simulink model "ball_and_beam"  (R2020b)
settings: Solver=VariableStepAuto  StartTime=0.0  StopTime=10.0  RelTol=1e-3
values from neighbouring files (symbols this model uses):
  h = 0.01    [main_ball_and_beam_dlqr.m]
  setpoint = -0.5    [main_ball_and_beam_dlqr.m]
  X0 = [0; 0; 0; 0]    [main_ball_and_beam_dlqr.m]
undefined symbols (not defined in the file or in its folder): add_states, lstates, ubar, xbar
libraries: cstblocks x1
settings Model: Creator=Kingdel  LastModifiedBy=mluser

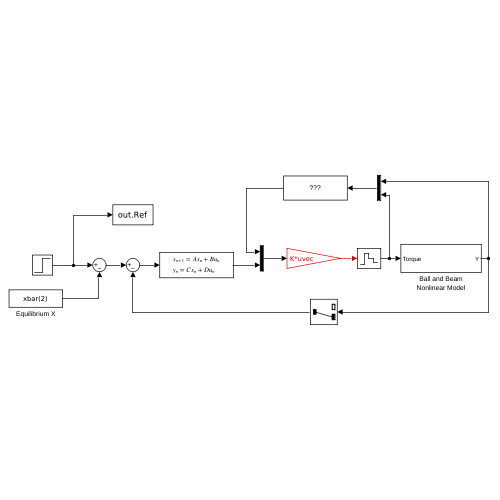
[thumbnail: Simulink's stored preview of the top-level diagram]
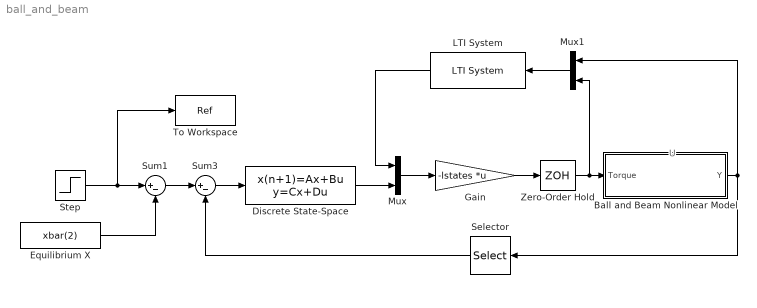
== system ball_and_beam ==
  note: U
  Ball and Beam Nonlinear Model : Subsystem
  Discrete State-Space : DiscreteStateSpace  A=add_states.A  B=add_states.B  C=eye(size(add_states.A))  D=zeros(size(add_states.B))  SampleTime=h
  Equilibrium X : Constant  Value=xbar(2)
  Gain : Gain  Gain=-lstates  Multiplication=Matrix(K*u) (u vector)  SampleTime=h
  LTI System : cstblocks/LTI System  sys=observer  IC=[]
  Mux : Mux  Inputs=2
  Mux1 : Mux  Inputs=2
  Selector : Selector  InputPortWidth=2  IndexOptions=Index vector (dialog)  Indices=2  OutputSizes=1
  Step : Step  Time=0  After=setpoint  SampleTime=h
  Sum1 : Sum  Inputs=|+-
  Sum3 : Sum  Inputs=|+-
  To Workspace : ToWorkspace  VariableName=Ref  SaveFormat=Structure With Time  SampleTime=h
  Zero-Order Hold : ZeroOrderHold  SampleTime=h
  wires:
  Gain/1 -> Zero-Order Hold/1
  Sum3/1 -> Discrete State-Space/1
  Discrete State-Space/1 -> Mux/2
  Mux/1 -> Gain/1
  Zero-Order Hold/1 -> Mux1/2, Ball and Beam Nonlinear Model/1(Torque)
  Step/1 -> To Workspace/1, Sum1/1
  Sum1/1 -> Sum3/1
  Equilibrium X/1 -> Sum1/2
  Ball and Beam Nonlinear Model/1(Y) -> Selector/1, Mux1/1
  Selector/1 -> Sum3/2
  Mux1/1 -> LTI System/1
  LTI System/1 -> Mux/1

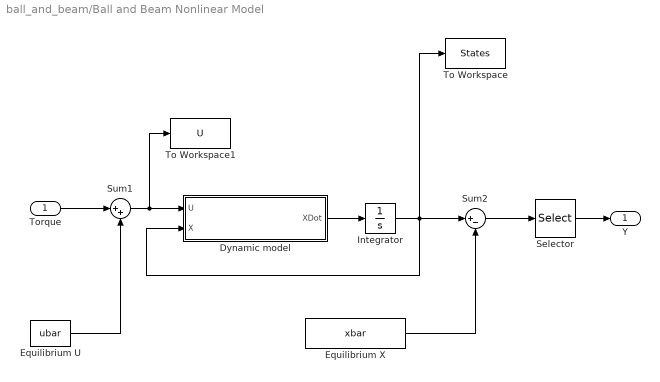
== system ball_and_beam/Ball and Beam Nonlinear Model ==
  Torque : Inport
  Dynamic model : MATLAB Function  TreatAsAtomicUnit=on
  Equilibrium U : Constant  Value=ubar
  Equilibrium X : Constant  Value=xbar
  Integrator : Integrator  InitialCondition=X0
  Selector : Selector  InputPortWidth=4  IndexOptions=Index vector (dialog)  Indices=[1,2]  OutputSizes=1
  Sum1 : Sum  Inputs=|++
  Sum2 : Sum  Inputs=|+-
  To Workspace : ToWorkspace  VariableName=States  SaveFormat=Structure With Time  SampleTime=h
  To Workspace1 : ToWorkspace  VariableName=U  SaveFormat=Structure With Time  SampleTime=h
  Y : Outport  VectorParamsAs1DForOutWhenUnconnected=off
  wires:
  Dynamic model/1(XDot) -> Integrator/1
  Integrator/1 -> To Workspace/1, Dynamic model/2(X), Sum2/1
  Selector/1 -> Y/1
  Equilibrium X/1 -> Sum2/2
  Sum2/1 -> Selector/1
  Equilibrium U/1 -> Sum1/2
  Torque/1 -> Sum1/1
  Sum1/1 -> Dynamic model/1(U), To Workspace1/1

== matlab function ball_and_beam/Ball and Beam Nonlinear Model/Dynamic model ==
  data: U input; XDot output; X input
function XDot = ball_and_beam_model(U,X)
%#codegen
% Constants of the model
[m,J,r,g]           = deal(0.1,0.025,0.01,9.807);

%% State space model
% x1 = theta, x2  = x, x3 = thetadot, x4 = xdot
[X1,X2,X3,X4]= deal(X(1),X(2),X(3),X(4));

% Inertia matrix
D           = [m*r^2+m*X2^2+J, -m*r; -m*r, m];

% Coriolis and centrifugal forces
H           = [2*m*X2*X4*X3; -m*X2*X3^2];

% Gravity forces
G           = [m*g*X2*cos(X1)-m*g*r*sin(X1); m*g*sin(X1)];

% Generalized effort
E           = [U; 0];

% Derivatives of states
XDot        = [X3; X4; D\(E-H-G)];
end
